simulink model "model"  (R2018a)
settings: Solver=VariableStepAuto  StartTime=0.0  StopTime=10.0  RelTol=1e-3
undefined symbols (not defined in the file): DegreePerSecond
libraries: simulink x2
settings Model: Creator=paul  LastModifiedBy=paul
settings SolverCC: ZeroCrossAlgorithm=Adaptive
settings DebuggingCC: MaxConsecutiveZCsMsg=none

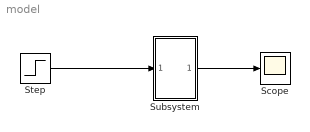
== system model ==
  Scope : Scope
  Step : Step  Time=0  After=250  SampleTime=0
  Subsystem : Subsystem  TreatAsAtomicUnit=on
  wires:
  Subsystem/1(Out1) -> Scope/1
  Step/1 -> Subsystem/1(PPM)

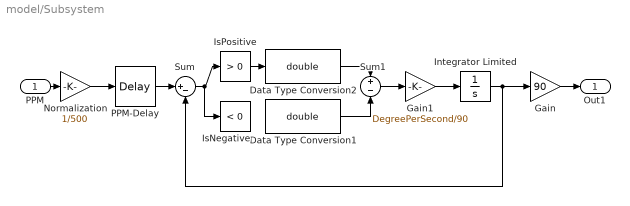
== system model/Subsystem ==
  PPM : Inport
  Data Type Conversion1 : DataTypeConversion  OutDataTypeStr=double
  Data Type Conversion2 : DataTypeConversion  OutDataTypeStr=double
  Gain : Gain  Gain=90
  Gain1 : Gain  Gain=DegreePerSecond/90
  Integrator Limited : Integrator  LimitOutput=on  UpperSaturationLimit=1  LowerSaturationLimit=-1
  IsNegative : simulink/Logic and Bit Operations/Compare To Zero  relop=<  OutDataTypeStr=boolean
  IsPositive : simulink/Logic and Bit Operations/Compare To Zero  relop=>  OutDataTypeStr=boolean
  Normalization : Gain  Gain=1/500
  PPM-Delay : TransportDelay  DelayTime=0.01
  Sum : Sum  Inputs=|+-
  Sum1 : Sum  Inputs=+|-
  Out1 : Outport
  wires:
  PPM/1 -> Normalization/1
  Normalization/1 -> PPM-Delay/1
  Gain1/1 -> Integrator Limited/1
  Gain/1 -> Out1/1
  PPM-Delay/1 -> Sum/1
  Integrator Limited/1 -> Sum/2, Gain/1
  IsPositive/1 -> Data Type Conversion2/1
  Sum/1 -> IsNegative/1, IsPositive/1
  Sum1/1 -> Gain1/1
  Data Type Conversion2/1 -> Sum1/1
  Data Type Conversion1/1 -> Sum1/2
